simulink model "model"  (R2019a)
settings: Solver=ode15s  StartTime=0.0  StopTime=tstop  MaxStep=1e-3  RelTol=1e-3  EnableMultiTasking=on
libraries: truetime x1
settings Model: Creator=The MathWorks, Inc.  LastModifiedBy=ramon
settings SolverCC: AlgebraicLoopSolver=LineSearch  MinimalZcImpactIntegration=on
settings DataIOCC: LimitDataPoints=on  SaveFormat=Array  ReturnWorkspaceOutputs=off
settings OptimizationCC: LifeSpan=inf
settings DebuggingCC: AlgebraicLoopMsg=none  UnderspecifiedInitializationDetection=Classic  MergeDetectMultiDrivingBlocksExec=none  SolverPrmCheckMsg=warning  AllowSymbolicDim=off  StateNameClashWarn=warning  SFUnexpectedBacktrackingDiag=warning  SFNoUnconditionalDefaultTransitionDiag=warning  SFExecutionAtInitializationDiag=none  ArithmeticOperatorsInVariantConditions=warning
settings HardwareCC: ProdBitPerPointer=32  ProdBitPerSizeT=32  ProdBitPerPtrDiffT=32  ProdLargestAtomicFloat=None  ProdIntDivRoundTo=Undefined  ProdEndianess=Unspecified  ProdWordSize=32  ProdHWDeviceType=32-bit Generic
settings ModelReferenceCC: PropagateSignalLabelsOutOfModel=off
settings SFSimCC: SimUseLocalCustomCode=off
settings RTWCC: RTWUseLocalCustomCode=off
settings CodeAppCC: StateflowObjectComments=on
settings GRTTargetCC: TargetLangStandard=C89/C90 (ANSI)
settings ConfigComp: CovMetricSettings=dw  CovSaveCumulativeToWorkspaceVar=on  CovSaveSingleToWorkspaceVar=on  CovExternalEMLEnable=off  CovSFcnEnable=off
settings SimscapeCC: SimscapeNormalizeSystem=off

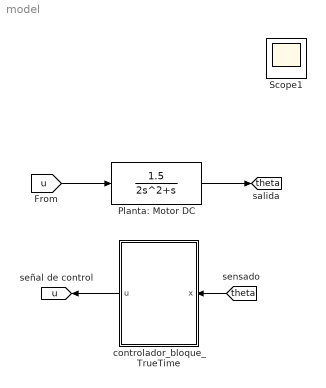
== system model ==
  Planta: Motor DC : TransferFcn  Numerator=[1.5]  Denominator=[2 1 0]
  controlador_bloque_TrueTime : Subsystem
  Scope1 : Scope
  tag scope: theta=global, u=global
  wires:
  controlador_bloque_TrueTime/1(u) -> [u]
  [theta] -> controlador_bloque_TrueTime/1(x)
  [u] -> Planta: Motor DC/1
  Planta: Motor DC/1 -> [theta]

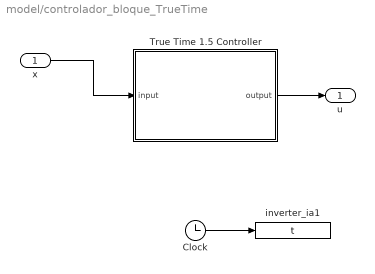
== system model/controlador_bloque_TrueTime ==
  x : Inport
  Clock : Clock
  True Time 1.5 Controller : Subsystem
      mask Display: plot([0 20 20 30 30 40 40 55], [5 5 25 25 15 15 12 12])
  inverter_ia1 : ToWorkspace  VariableName=t  SampleTime=-1
  u : Outport  VectorParamsAs1DForOutWhenUnconnected=off
  wires:
  Clock/1 -> inverter_ia1/1
  x/1 -> True Time 1.5 Controller/1(input)
  True Time 1.5 Controller/1(output) -> u/1

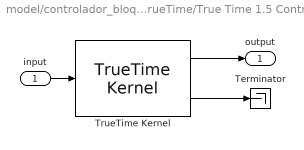
== system model/controlador_bloque_TrueTime/True Time 1.5 Controller ==
  input : Inport
  Terminator : Terminator
  TrueTime Kernel : truetime/TrueTime Kernel  sfun=simulator_init  args=[]  ninputsoutputs=[1 1]  ntriggers=0  trigtype=rising  nwnodenbr=[]  clockoffsetdrift=[0 0]  schedoutput=on  battery=off  poweroutput=off
  output : Outport  VectorParamsAs1DForOutWhenUnconnected=off
  wires:
  input/1 -> TrueTime Kernel/1
  TrueTime Kernel/2 -> Terminator/1
  TrueTime Kernel/1 -> output/1
